simulink model "controlledheatflow"  (R2021a)
settings: Solver=VariableStepAuto  StartTime=0.0  StopTime=60*60*12  RelTol=1e-3
model workspace (MAT data in the model file):
  Dwindow = 2700
  Hroom = 4
  Hwindow = 1.8
  LWindow = 0.01
  Lroom = 30
  M_air = 1470
  Wroom = 10
  Wwindow = 2.4
  c_air = 1005.4
  c_window = 840
  h_A_Wnd = 25
  h_Wnd_Atm = 32
  kWindow = 0.78
  windowArea = 4.32
  windowMass = 116.64
libraries: fl_lib x12, nesl_utility x3
settings Model: Creator=IT-Defenders  LastModifiedBy=IT-Defenders

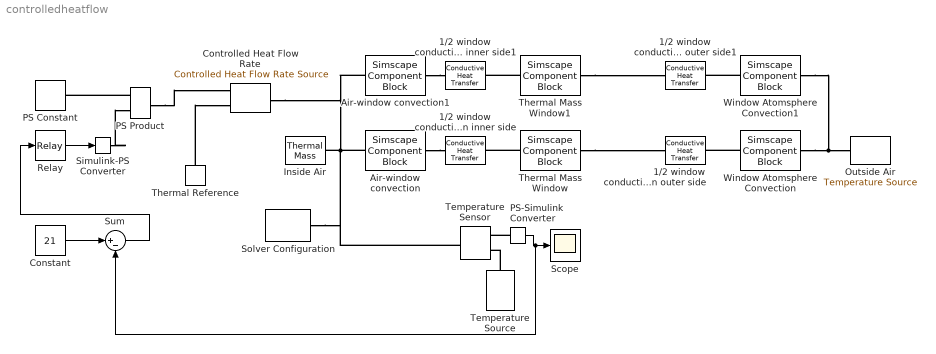
== system controlledheatflow ==
  1/2 window conduction inner side : fl_lib/Thermal/Thermal Elements/Conductive Heat Transfer  area=windowArea m^2  thickness=LWindow/2 m  th_cond=kWindow W/(m*K)  T_specify=off  T_priority=None  T=0 K  T_nominal_specify=off  T_nominal_unit=K  T_nominal_value=1  Q_specify=off  Q_priority=None  Q=0 W  Q_nominal_specify=off  Q_nominal_unit=W  Q_nominal_value=1
  1/2 window conduction inner side1 : fl_lib/Thermal/Thermal Elements/Conductive Heat Transfer  area=windowArea m^2  thickness=LWindow/2 m  th_cond=kWindow W/(m*K)  T_specify=off  T_priority=None  T=0 K  T_nominal_specify=off  T_nominal_unit=K  T_nominal_value=1  Q_specify=off  Q_priority=None  Q=0 W  Q_nominal_specify=off  Q_nominal_unit=W  Q_nominal_value=1
  1/2 window conduction outer side : fl_lib/Thermal/Thermal Elements/Conductive Heat Transfer  area=windowArea m^2  thickness=LWindow/2 m  th_cond=kWindow W/(m*K)  T_specify=off  T_priority=None  T=0 K  T_nominal_specify=off  T_nominal_unit=K  T_nominal_value=1  Q_specify=off  Q_priority=None  Q=0 W  Q_nominal_specify=off  Q_nominal_unit=W  Q_nominal_value=1
  1/2 window conduction outer side1 : fl_lib/Thermal/Thermal Elements/Conductive Heat Transfer  area=windowArea m^2  thickness=LWindow/2 m  th_cond=kWindow W/(m*K)  T_specify=off  T_priority=None  T=0 K  T_nominal_specify=off  T_nominal_unit=K  T_nominal_value=1  Q_specify=off  Q_priority=None  Q=0 W  Q_nominal_specify=off  Q_nominal_unit=W  Q_nominal_value=1
  Air-window convection : SimscapeComponentBlock  SourceFile=convection  ComponentPath=convection  ComponentVariants="[\"convection\"]"  ComponentVariantNames="[\"convection\"]"  ClassName=convection  SchemaVersion=1  thermal_type=foundation.enum.constant_variable.constant  area=windowArea m^2  heat_tr_coeff=h_A_Wnd W/(m^2 * K)  min_heat_tr_coeff=1e-3 W/(m^2 * K)  T_specify=off  T_priority=None  T=0 K  T_nominal_specify=off  T_nominal_unit=K  T_nominal_value=1  Q_specify=off  Q_priority=None  Q=0 W  Q_nominal_specify=off  Q_nominal_unit=W  Q_nominal_value=1
      settings: CopyFcn=simscape.engine.sli.internal.componentblockcallback(gcbh,'COPY')  PreCopyFcn=simscape.engine.sli.internal.componentblockcallback(gcbh,'PRECOPY')  PreDeleteFcn=simscape.engine.sli.internal.componentblockcallback(gcbh,'PREDELETE')  InternalSimscapePortConfiguration="{\"Bottom\":[],\"Left\":[{\"id\":\"A\",\"label\":\"A\",\"type\":\"foundation.thermal.thermal\"}],\"Right\":[{\"id\":\"B\",\"label\":\"B\",\"type\":\"foundation.thermal.thermal\"}],\"Top\":[]}"
      mask Type: Convective Heat Transfer
  Air-window convection1 : SimscapeComponentBlock  SourceFile=convection  ComponentPath=convection  ComponentVariants="[\"convection\"]"  ComponentVariantNames="[\"convection\"]"  ClassName=convection  SchemaVersion=1  thermal_type=foundation.enum.constant_variable.constant  area=windowArea m^2  heat_tr_coeff=h_A_Wnd W/(m^2 * K)  min_heat_tr_coeff=1e-3 W/(m^2 * K)  T_specify=off  T_priority=None  T=0 K  T_nominal_specify=off  T_nominal_unit=K  T_nominal_value=1  Q_specify=off  Q_priority=None  Q=0 W  Q_nominal_specify=off  Q_nominal_unit=W  Q_nominal_value=1
      settings: CopyFcn=simscape.engine.sli.internal.componentblockcallback(gcbh,'COPY')  PreCopyFcn=simscape.engine.sli.internal.componentblockcallback(gcbh,'PRECOPY')  PreDeleteFcn=simscape.engine.sli.internal.componentblockcallback(gcbh,'PREDELETE')  InternalSimscapePortConfiguration="{\"Bottom\":[],\"Left\":[{\"id\":\"A\",\"label\":\"A\",\"type\":\"foundation.thermal.thermal\"}],\"Right\":[{\"id\":\"B\",\"label\":\"B\",\"type\":\"foundation.thermal.thermal\"}],\"Top\":[]}"
      mask Type: Convective Heat Transfer
  Constant : Constant  Value=21
  "Controlled Heat Flow Rate " : fl_lib/Thermal/Thermal Sources/Controlled Heat Flow Rate Source
  Inside Air : fl_lib/Thermal/Thermal Elements/Thermal Mass  mass=M_air kg  sp_heat=c_air J/kg/K  T_specify=on  T_priority=High  T=20 degC  T_nominal_specify=off  T_nominal_unit=K  T_nominal_value=1  Q_specify=off  Q_priority=None  Q=0 W  Q_nominal_specify=off  Q_nominal_unit=W  Q_nominal_value=1
  Outside Air : fl_lib/Thermal/Thermal Sources/Temperature Source  temperature=-6 degC
  PS Constant : fl_lib/Physical Signals/Sources/PS Constant  constant=17000 J/s
  PS Product : fl_lib/Physical Signals/Functions/PS Product
  PS-Simulink Converter : nesl_utility/PS-Simulink Converter  PhysicalDomain=network_engine_domain  SubClassName=ps_output  LeftPortType=input  RightPortType=output  PseudoPeriodic=off  Frequencies=[]  Unit=inherit  AffineConversion=off
      settings: SourceProductBaseCode=PW,SS
  Relay : Relay  OnSwitchValue=1  OffSwitchValue=-1
  Scope : Scope
  Simulink-PS Converter : nesl_utility/Simulink-PS Converter  PhysicalDomain=network_engine_domain  SubClassName=ps_input  LeftPortType=input  RightPortType=output  PseudoPeriodic=off  Frequencies=[]  NoiseDistribution=none  NoiseParameters=[]  Unit=1  AffineConversion=off  FilteringAndDerivatives=provide  SimscapeFilterOrder=1  InputFilterTimeConstant=0.001  UdotUserProvided=0
      settings: SourceProductBaseCode=PW,SS
  Solver Configuration : nesl_utility/Solver Configuration  PhysicalDomain=network_engine_domain  SubClassName=solver  LeftPortType=input  RightPortType=generic  Tones=[]  Harmonics=[]  SimulateNoise=off  Profile=off  UseLocalSampling=off  EnableSwitchedLinearOptims=on  FrequencyDomain=off  UseCCode=off  RelTol=0.001  AbsTol=1e-06  MinStep=1e-09  ToWorkspace=off  RevertToSquareIcSolve=off  NumHomotopyIterations=100  PhasorMode=off  PhasorModeNumHarmonics=1  DoDC=off  ResidualTolerance=1e-09  UseLocalSolver=off  LocalSolverChoice=NE_BACKWARD_EULER_ADVANCER  LocalSolverSampleTime=0.001  DoFixedCost=off  MaxNonlinIter=3  MaxModeIter=2  ComputeImpulses=off  ImpulseIterations=2  LinearAlgebra=auto  EquationFormulation=NE_TIME_EF  DelaysMemoryBudget=1024  AutomaticFiltering=on  FilteringTimeConstant=0.001  PartitionStorageMethod=AS_NEEDED  PartitionMemoryBudget=1024  PartitionMethod=ROBUST
      settings: SourceProductBaseCode=PW,SS
  Sum : Sum  Inputs=|+-
  Temperature Sensor : fl_lib/Thermal/Thermal Sensors/Temperature Sensor
  Temperature Source : fl_lib/Thermal/Thermal Sources/Temperature Source  temperature=0 degC
  Thermal Mass Window : SimscapeComponentBlock  SourceFile=mass  ComponentPath=mass  ComponentVariants="[\"mass\"]"  ComponentVariantNames="[\"mass\"]"  ClassName=mass  SchemaVersion=1  mass_type=foundation.enum.constant_variable.constant  mass=windowMass kg  sp_heat=c_window J/kg/K  mass_min=1e-6 kg  num_ports=foundation.enum.numPorts2.two  m_specify=off  m_priority=High  m=1 kg  m_nominal_specify=off  m_nominal_unit=kg  m_nominal_value=1  T_specify=on  T_priority=High  T=10 degC  T_nominal_specify=off  T_nominal_unit=K  T_nominal_value=1  Q_specify=off  Q_priority=None  Q=0 W  Q_nominal_specify=off  Q_nominal_unit=W  Q_nominal_value=1
      settings: CopyFcn=simscape.engine.sli.internal.componentblockcallback(gcbh,'COPY')  PreCopyFcn=simscape.engine.sli.internal.componentblockcallback(gcbh,'PRECOPY')  PreDeleteFcn=simscape.engine.sli.internal.componentblockcallback(gcbh,'PREDELETE')  InternalSimscapePortConfiguration="{\"Bottom\":[],\"Left\":[{\"id\":\"M\",\"label\":\"\",\"type\":\"foundation.thermal.thermal\"}],\"Right\":[{\"id\":\"N\",\"label\":\"\",\"type\":\"foundation.thermal.thermal\"}],\"Top\":[]}"
      mask Type: Thermal Mass
  Thermal Mass Window1 : SimscapeComponentBlock  SourceFile=mass  ComponentPath=mass  ComponentVariants="[\"mass\"]"  ComponentVariantNames="[\"mass\"]"  ClassName=mass  SchemaVersion=1  mass_type=foundation.enum.constant_variable.constant  mass=windowMass kg  sp_heat=c_window J/kg/K  mass_min=1e-6 kg  num_ports=foundation.enum.numPorts2.two  m_specify=off  m_priority=High  m=1 kg  m_nominal_specify=off  m_nominal_unit=kg  m_nominal_value=1  T_specify=on  T_priority=High  T=10 degC  T_nominal_specify=off  T_nominal_unit=K  T_nominal_value=1  Q_specify=off  Q_priority=None  Q=0 W  Q_nominal_specify=off  Q_nominal_unit=W  Q_nominal_value=1
      settings: CopyFcn=simscape.engine.sli.internal.componentblockcallback(gcbh,'COPY')  PreCopyFcn=simscape.engine.sli.internal.componentblockcallback(gcbh,'PRECOPY')  PreDeleteFcn=simscape.engine.sli.internal.componentblockcallback(gcbh,'PREDELETE')  InternalSimscapePortConfiguration="{\"Bottom\":[],\"Left\":[{\"id\":\"M\",\"label\":\"\",\"type\":\"foundation.thermal.thermal\"}],\"Right\":[{\"id\":\"N\",\"label\":\"\",\"type\":\"foundation.thermal.thermal\"}],\"Top\":[]}"
      mask Type: Thermal Mass
  Thermal Reference : fl_lib/Thermal/Thermal Elements/Thermal Reference
  Window Atomsphere Convection : SimscapeComponentBlock  SourceFile=convection  ComponentPath=convection  ComponentVariants="[\"convection\"]"  ComponentVariantNames="[\"convection\"]"  ClassName=convection  SchemaVersion=1  thermal_type=foundation.enum.constant_variable.constant  area=windowArea m^2  heat_tr_coeff=h_Wnd_Atm W/(m^2 * K)  min_heat_tr_coeff=1e-3 W/(m^2 * K)  T_specify=off  T_priority=None  T=0 K  T_nominal_specify=off  T_nominal_unit=K  T_nominal_value=1  Q_specify=off  Q_priority=None  Q=0 W  Q_nominal_specify=off  Q_nominal_unit=W  Q_nominal_value=1
      settings: CopyFcn=simscape.engine.sli.internal.componentblockcallback(gcbh,'COPY')  PreCopyFcn=simscape.engine.sli.internal.componentblockcallback(gcbh,'PRECOPY')  PreDeleteFcn=simscape.engine.sli.internal.componentblockcallback(gcbh,'PREDELETE')  InternalSimscapePortConfiguration="{\"Bottom\":[],\"Left\":[{\"id\":\"A\",\"label\":\"A\",\"type\":\"foundation.thermal.thermal\"}],\"Right\":[{\"id\":\"B\",\"label\":\"B\",\"type\":\"foundation.thermal.thermal\"}],\"Top\":[]}"
      mask Type: Convective Heat Transfer
  Window Atomsphere Convection1 : SimscapeComponentBlock  SourceFile=convection  ComponentPath=convection  ComponentVariants="[\"convection\"]"  ComponentVariantNames="[\"convection\"]"  ClassName=convection  SchemaVersion=1  thermal_type=foundation.enum.constant_variable.constant  area=windowArea m^2  heat_tr_coeff=h_Wnd_Atm W/(m^2 * K)  min_heat_tr_coeff=1e-3 W/(m^2 * K)  T_specify=off  T_priority=None  T=0 K  T_nominal_specify=off  T_nominal_unit=K  T_nominal_value=1  Q_specify=off  Q_priority=None  Q=0 W  Q_nominal_specify=off  Q_nominal_unit=W  Q_nominal_value=1
      settings: CopyFcn=simscape.engine.sli.internal.componentblockcallback(gcbh,'COPY')  PreCopyFcn=simscape.engine.sli.internal.componentblockcallback(gcbh,'PRECOPY')  PreDeleteFcn=simscape.engine.sli.internal.componentblockcallback(gcbh,'PREDELETE')  InternalSimscapePortConfiguration="{\"Bottom\":[],\"Left\":[{\"id\":\"A\",\"label\":\"A\",\"type\":\"foundation.thermal.thermal\"}],\"Right\":[{\"id\":\"B\",\"label\":\"B\",\"type\":\"foundation.thermal.thermal\"}],\"Top\":[]}"
      mask Type: Convective Heat Transfer
  wires:
  PS-Simulink Converter/1 -> Sum/2, Scope/1
  Constant/1 -> Sum/1
  Sum/1 -> Relay/1
  Relay/1 -> Simulink-PS Converter/1
  connections:
  Air-window convection/LConn1 -- Air-window convection1/LConn1 -- "Controlled Heat Flow Rate "/LConn1 -- Inside Air/LConn1 -- Temperature Sensor/LConn1 -- Solver Configuration/RConn1
  Thermal Mass Window/RConn1 -- 1/2 window conduction outer side/LConn1
  Thermal Mass Window/LConn1 -- 1/2 window conduction inner side/RConn1
  Air-window convection/RConn1 -- 1/2 window conduction inner side/LConn1
  Window Atomsphere Convection/LConn1 -- 1/2 window conduction outer side/RConn1
  Window Atomsphere Convection/RConn1 -- Window Atomsphere Convection1/RConn1 -- Outside Air/LConn1
  Temperature Source/LConn1 -- Temperature Sensor/RConn1
  PS-Simulink Converter/LConn1 -- Temperature Sensor/RConn2
  Thermal Reference/LConn1 -- "Controlled Heat Flow Rate "/RConn2
  PS Product/LConn1 -- PS Constant/RConn1
  Simulink-PS Converter/RConn1 -- PS Product/LConn2
  PS Product/RConn1 -- "Controlled Heat Flow Rate "/RConn1
  Window Atomsphere Convection1/LConn1 -- 1/2 window conduction outer side1/RConn1
  Air-window convection1/RConn1 -- 1/2 window conduction inner side1/LConn1
  Thermal Mass Window1/LConn1 -- 1/2 window conduction inner side1/RConn1
  Thermal Mass Window1/RConn1 -- 1/2 window conduction outer side1/LConn1
